simulink model "testmodel"  (R2025b)
settings: Solver=VariableStepAuto  StartTime=0.0  StopTime=2  RelTol=1e-3
values from neighbouring files (symbols this model uses):
  fs = 44100    [model.m]    (also in xgboost.m)
undefined symbols (not defined in the file or in its folder): c
libraries: audiofeatures x6, statsLibrary x3, deeplib x3, audiosources x1
settings Model: Creator=prashanth  LastModifiedBy=prashanth

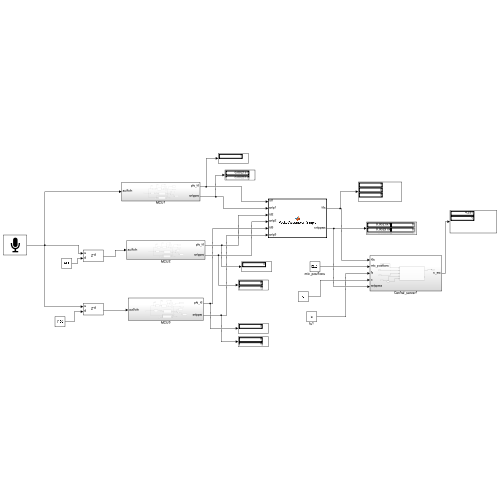
[thumbnail: Simulink's stored preview of the top-level diagram]
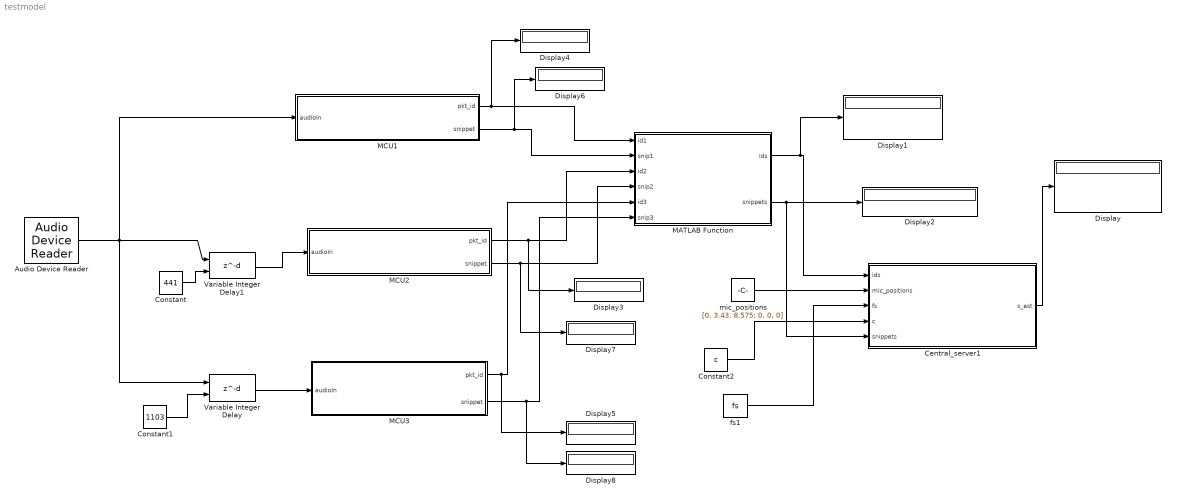
== system testmodel ==
  Audio Device Reader : audiosources/Audio Device Reader  Driver=CoreAudio  Device=Default  SampleRate=44100  NumChannels=1  SamplesPerFrame=44100  BitDepth=16-bit integer  NumBuffers=10  DefaultInputChannelMapping=on  InputChannelMapping=1:2  OutputNumOverrunSamples=off  OutputDataType=double  DriverIdx=5  DeviceWarnFlag=''
  Central_server1 : Subsystem
  Constant : Constant  Value=441
  Constant1 : Constant  Value=1103
  Constant2 : Constant  Value=c
  Display{,1..8} (9 alike) : Display
  MATLAB Function : MATLAB Function  TreatAsAtomicUnit=on
  MCU1 : Subsystem
  MCU2 : Subsystem
  MCU3 : Subsystem
  Variable Integer Delay : Delay  DelayLengthSource=Input port
      settings: InputPortMap=u0,p1
  Variable Integer Delay1 : Delay  DelayLengthSource=Input port
      settings: InputPortMap=u0,p1
  fs1 : Constant  Value=fs
  mic_positions : Constant  Value=[0, 3.43, 8.575; 0, 0, 0]
  wires:
  Audio Device Reader/1 -> MCU1/1(audioIn), Variable Integer Delay1/1, Variable Integer Delay/1
  Variable Integer Delay1/1 -> MCU2/1(audioIn)
  Variable Integer Delay/1 -> MCU3/1(audioIn)
  Constant/1 -> Variable Integer Delay1/2
  Constant1/1 -> Variable Integer Delay/2
  MCU1/1(pkt_id) -> Display4/1, MATLAB Function/1(id1)
  MCU1/2(snippet) -> Display6/1, MATLAB Function/2(snip1)
  MCU3/1(pkt_id) -> Display5/1, MATLAB Function/5(id3)
  MCU3/2(snippet) -> Display8/1, MATLAB Function/6(snip3)
  MATLAB Function/1(ids) -> Display1/1, Central_server1/1(ids)
  fs1/1 -> Central_server1/3(fs)
  mic_positions/1 -> Central_server1/2(mic_positions)
  Constant2/1 -> Central_server1/4(c)
  Central_server1/1(s_est) -> Display/1
  MATLAB Function/2(snippets) -> Central_server1/5(snippets), Display2/1
  MCU2/1(pkt_id) -> Display3/1, MATLAB Function/3(id2)
  MCU2/2(snippet) -> Display7/1, MATLAB Function/4(snip2)

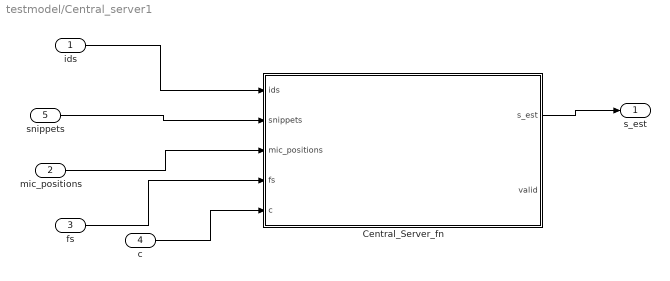
== system testmodel/Central_server1 ==
  ids : Inport
  mic_positions : Inport  Port=2
  fs : Inport  Port=3
  c : Inport  Port=4
  snippets : Inport  Port=5
  Central_Server_fn : MATLAB Function  TreatAsAtomicUnit=on
  s_est : Outport
  wires:
  Central_Server_fn/1(s_est) -> s_est/1
  ids/1 -> Central_Server_fn/1(ids)
  mic_positions/1 -> Central_Server_fn/3(mic_positions)
  fs/1 -> Central_Server_fn/4(fs)
  c/1 -> Central_Server_fn/5(c)
  snippets/1 -> Central_Server_fn/2(snippets)

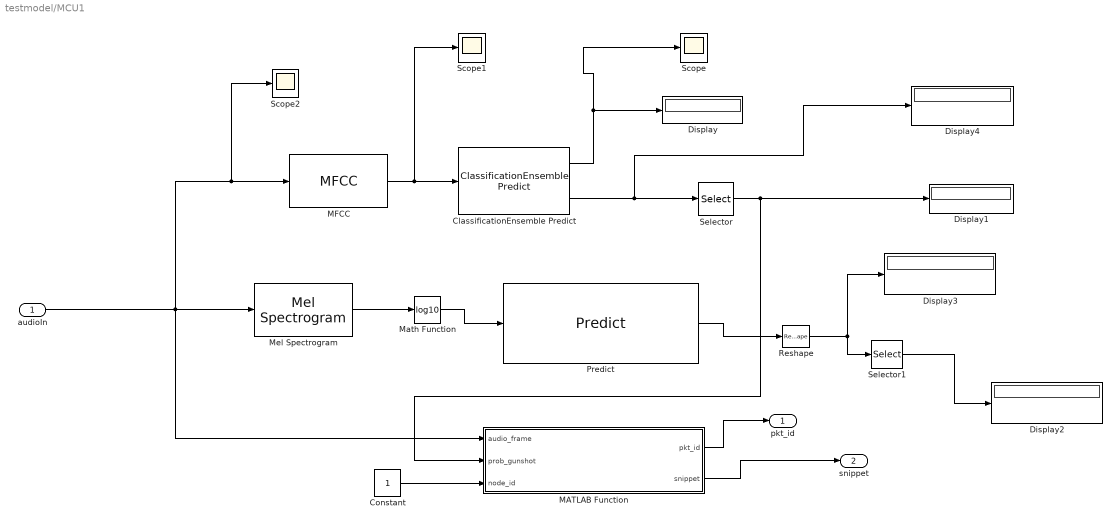
== system testmodel/MCU1 ==
  audioIn : Inport
  ClassificationEnsemble Predict : statsLibrary/Classification/ClassificationEnsemble Predict  TrainedLearner=trainedModel  ShowOutputScore=on  LabelOutMin=[]  LabelOutMax=[]  ScoreOutMin=[]  ScoreOutMax=[]  RawScoreOutMin=[]  RawScoreOutMax=[]  WeakLearnerOutMin=[]  WeakLearnerOutMax=[]  StoredEnumName=trainedModel_enumLabels
  Constant : Constant
  Display{,1..4} (5 alike) : Display
  MATLAB Function : MATLAB Function  TreatAsAtomicUnit=on
  MFCC : audiofeatures/MFCC  WindowParameter=hamming(1024,'periodic')  OverlapLength=512  NumCoeffs=13  Rectification=Logarithm  AppendDelta=on  AppendDeltaDelta=off  DeltaWindowLength=9  NumFeatureVectors=1  NumFeatureVectorOverlap=0  InheritSampleRate=on  SampleRate=44.1e3  NumBands=32  AutoFrequencyRange=on  FrequencyRange=[0, 22050]  FilterBankDesignDomain=linear  FilterBankNormalization=bandwidth  MelStyle=oshaughnessy  WindowNormalization=on  SpectrumType=power  AutoFFTLength=on  FFTLength=1024
  Math Function : Math  Operator=log10
  Mel Spectrogram : audiofeatures/Mel Spectrogram  FrequencyScale=mel  AutoNumBands=off  NumBands=32  AutoFrequencyRange=on  FrequencyRange=[0, 22050]  FilterBankDesignDomain=linear  FilterBankNormalization=bandwidth  MelStyle=oshaughnessy  OutputFrequencyVector=off  WindowParameter=hamming(1024,'periodic')  WindowNormalization=on  OverlapLength=512  AutoFFTLength=on  FFTLength=1024  SpectrumType=magnitude  ApplyLog=off  NumHops=85  NumHopsOverlap=0  InheritSampleRate=on  SampleRate=44.1e3
  Predict : deeplib/Predict  Network=Network from MAT-file  NetworkFunction=squeezenet  NetworkFilePath=/Users/prashanth/Desktop/karthik/gunshotCNN.mat  MiniBatchSize=128  InputDataFormats={'',''}  Predictions=off  Activations={'softmax'}  ForceInterpretedSim=off  EnableDLNetwork=on  LastKnownNetworkFilePath=''  LastKnownNetworkTimeStamp=''
  Reshape : Reshape
  Scope : Scope
      settings: ActiveDisplayYMinimum=-1  ActiveDisplayYMaximum=1
  Scope1 : Scope
      settings: ActiveDisplayYMinimum=-2027.6320329799446  ActiveDisplayYMaximum=845.22597661163
  Scope2 : Scope
      settings: ActiveDisplayYMinimum=-0.30791958580274859  ActiveDisplayYMaximum=0.10660759871682185  DataLoggingVariableName=ScopeData2
  Selector : Selector  InputPortWidth=2  IndexOptions=Index vector (dialog)  Indices=1  OutputSizes=1
  Selector1 : Selector  InputPortWidth=2  IndexOptions=Index vector (dialog)  Indices=1  OutputSizes=1
  pkt_id : Outport
  snippet : Outport  Port=2
  wires:
  Selector/1 -> MATLAB Function/2(prob_gunshot), Display1/1
  Reshape/1 -> Selector1/1, Display3/1
  MFCC/1 -> Scope1/1, ClassificationEnsemble Predict/1
  Predict/1 -> Reshape/1
  Mel Spectrogram/1 -> Math Function/1
  Selector1/1 -> Display2/1
  Math Function/1 -> Predict/1
  audioIn/1 -> MATLAB Function/1(audio_frame), Mel Spectrogram/1, MFCC/1, Scope2/1
  ClassificationEnsemble Predict/2 -> Display4/1, Selector/1
  ClassificationEnsemble Predict/1 -> Scope/1, Display/1
  Constant/1 -> MATLAB Function/3(node_id)
  MATLAB Function/1(pkt_id) -> pkt_id/1
  MATLAB Function/2(snippet) -> snippet/1

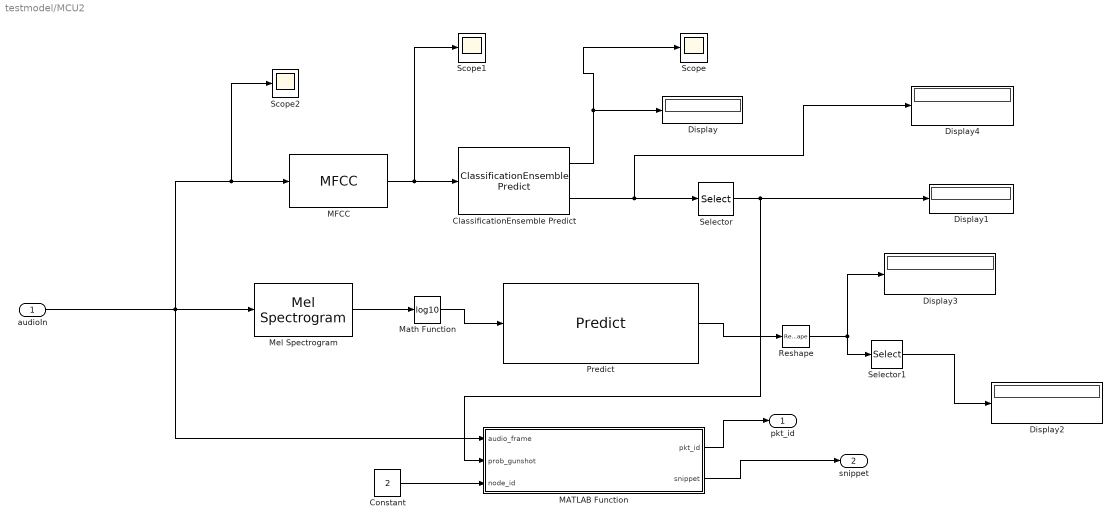
== system testmodel/MCU2 ==
  audioIn : Inport
  ClassificationEnsemble Predict : statsLibrary/Classification/ClassificationEnsemble Predict  TrainedLearner=trainedModel  ShowOutputScore=on  LabelOutMin=[]  LabelOutMax=[]  ScoreOutMin=[]  ScoreOutMax=[]  RawScoreOutMin=[]  RawScoreOutMax=[]  WeakLearnerOutMin=[]  WeakLearnerOutMax=[]  StoredEnumName=trainedModel_enumLabels
  Constant : Constant  Value=2
  Display{,1..4} (5 alike) : Display
  MATLAB Function : MATLAB Function  TreatAsAtomicUnit=on
  MFCC : audiofeatures/MFCC  WindowParameter=hamming(1024,'periodic')  OverlapLength=512  NumCoeffs=13  Rectification=Logarithm  AppendDelta=on  AppendDeltaDelta=off  DeltaWindowLength=9  NumFeatureVectors=1  NumFeatureVectorOverlap=0  InheritSampleRate=on  SampleRate=44.1e3  NumBands=32  AutoFrequencyRange=on  FrequencyRange=[0, 22050]  FilterBankDesignDomain=linear  FilterBankNormalization=bandwidth  MelStyle=oshaughnessy  WindowNormalization=on  SpectrumType=power  AutoFFTLength=on  FFTLength=1024
  Math Function : Math  Operator=log10
  Mel Spectrogram : audiofeatures/Mel Spectrogram  FrequencyScale=mel  AutoNumBands=off  NumBands=32  AutoFrequencyRange=on  FrequencyRange=[0, 22050]  FilterBankDesignDomain=linear  FilterBankNormalization=bandwidth  MelStyle=oshaughnessy  OutputFrequencyVector=off  WindowParameter=hamming(1024,'periodic')  WindowNormalization=on  OverlapLength=512  AutoFFTLength=on  FFTLength=1024  SpectrumType=magnitude  ApplyLog=off  NumHops=85  NumHopsOverlap=0  InheritSampleRate=on  SampleRate=44.1e3
  Predict : deeplib/Predict  Network=Network from MAT-file  NetworkFunction=squeezenet  NetworkFilePath=/Users/prashanth/Desktop/karthik/gunshotCNN.mat  MiniBatchSize=128  InputDataFormats={'',''}  Predictions=off  Activations={'softmax'}  ForceInterpretedSim=off  EnableDLNetwork=on  LastKnownNetworkFilePath=''  LastKnownNetworkTimeStamp=''
  Reshape : Reshape
  Scope : Scope
      settings: ActiveDisplayYMinimum=0.875  ActiveDisplayYMaximum=2.125  DataLoggingVariableName=ScopeData3
  Scope1 : Scope
      settings: ActiveDisplayYMinimum=-2027.6320329799446  ActiveDisplayYMaximum=845.22597661163  DataLoggingVariableName=ScopeData4
  Scope2 : Scope
      settings: ActiveDisplayYMinimum=-0.30791958580274859  ActiveDisplayYMaximum=0.10660759871682185  DataLoggingVariableName=ScopeData5
  Selector : Selector  InputPortWidth=2  IndexOptions=Index vector (dialog)  Indices=1  OutputSizes=1
  Selector1 : Selector  InputPortWidth=2  IndexOptions=Index vector (dialog)  Indices=1  OutputSizes=1
  pkt_id : Outport
  snippet : Outport  Port=2
  wires:
  Mel Spectrogram/1 -> Math Function/1
  Math Function/1 -> Predict/1
  ClassificationEnsemble Predict/2 -> Display4/1, Selector/1
  Constant/1 -> MATLAB Function/3(node_id)
  ClassificationEnsemble Predict/1 -> Scope/1, Display/1
  MATLAB Function/1(pkt_id) -> pkt_id/1
  Predict/1 -> Reshape/1
  Selector1/1 -> Display2/1
  Reshape/1 -> Selector1/1, Display3/1
  MFCC/1 -> Scope1/1, ClassificationEnsemble Predict/1
  MATLAB Function/2(snippet) -> snippet/1
  Selector/1 -> MATLAB Function/2(prob_gunshot), Display1/1
  audioIn/1 -> MATLAB Function/1(audio_frame), Mel Spectrogram/1, MFCC/1, Scope2/1

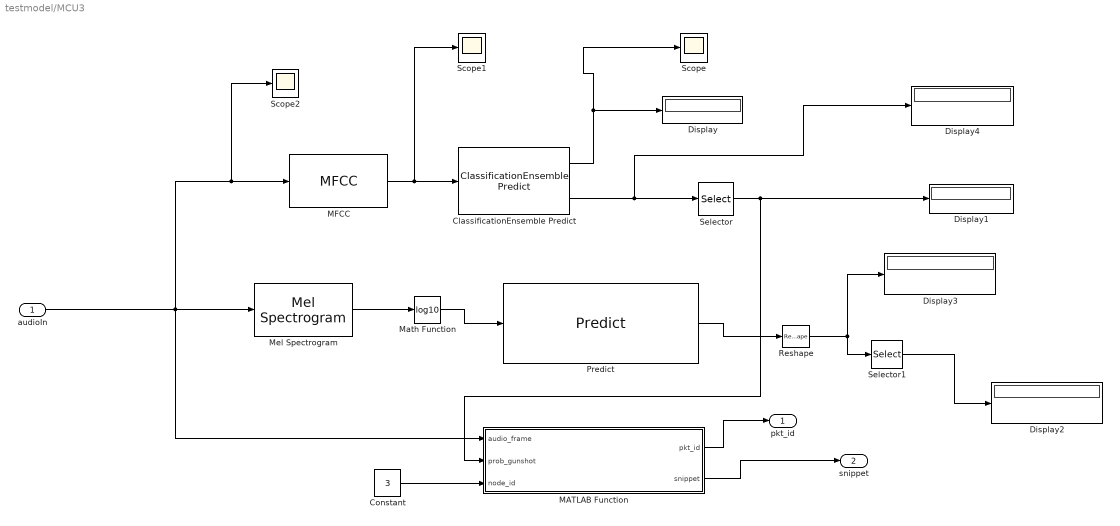
== system testmodel/MCU3 ==
  audioIn : Inport
  ClassificationEnsemble Predict : statsLibrary/Classification/ClassificationEnsemble Predict  TrainedLearner=trainedModel  ShowOutputScore=on  LabelOutMin=[]  LabelOutMax=[]  ScoreOutMin=[]  ScoreOutMax=[]  RawScoreOutMin=[]  RawScoreOutMax=[]  WeakLearnerOutMin=[]  WeakLearnerOutMax=[]  StoredEnumName=trainedModel_enumLabels
  Constant : Constant  Value=3
  Display{,1..4} (5 alike) : Display
  MATLAB Function : MATLAB Function  TreatAsAtomicUnit=on
  MFCC : audiofeatures/MFCC  WindowParameter=hamming(1024,'periodic')  OverlapLength=512  NumCoeffs=13  Rectification=Logarithm  AppendDelta=on  AppendDeltaDelta=off  DeltaWindowLength=9  NumFeatureVectors=1  NumFeatureVectorOverlap=0  InheritSampleRate=on  SampleRate=44.1e3  NumBands=32  AutoFrequencyRange=on  FrequencyRange=[0, 22050]  FilterBankDesignDomain=linear  FilterBankNormalization=bandwidth  MelStyle=oshaughnessy  WindowNormalization=on  SpectrumType=power  AutoFFTLength=on  FFTLength=1024
  Math Function : Math  Operator=log10
  Mel Spectrogram : audiofeatures/Mel Spectrogram  FrequencyScale=mel  AutoNumBands=off  NumBands=32  AutoFrequencyRange=on  FrequencyRange=[0, 22050]  FilterBankDesignDomain=linear  FilterBankNormalization=bandwidth  MelStyle=oshaughnessy  OutputFrequencyVector=off  WindowParameter=hamming(1024,'periodic')  WindowNormalization=on  OverlapLength=512  AutoFFTLength=on  FFTLength=1024  SpectrumType=magnitude  ApplyLog=off  NumHops=85  NumHopsOverlap=0  InheritSampleRate=on  SampleRate=44.1e3
  Predict : deeplib/Predict  Network=Network from MAT-file  NetworkFunction=squeezenet  NetworkFilePath=/Users/prashanth/Desktop/karthik/gunshotCNN.mat  MiniBatchSize=128  InputDataFormats={'',''}  Predictions=off  Activations={'softmax'}  ForceInterpretedSim=off  EnableDLNetwork=on  LastKnownNetworkFilePath=''  LastKnownNetworkTimeStamp=''
  Reshape : Reshape
  Scope : Scope
      settings: ActiveDisplayYMinimum=0.875  ActiveDisplayYMaximum=2.125  DataLoggingVariableName=ScopeData6
  Scope1 : Scope
      settings: ActiveDisplayYMinimum=-2027.6320329799446  ActiveDisplayYMaximum=845.22597661163  DataLoggingVariableName=ScopeData7
  Scope2 : Scope
      settings: ActiveDisplayYMinimum=-0.30791958580274859  ActiveDisplayYMaximum=0.10660759871682185  DataLoggingVariableName=ScopeData8
  Selector : Selector  InputPortWidth=2  IndexOptions=Index vector (dialog)  Indices=1  OutputSizes=1
  Selector1 : Selector  InputPortWidth=2  IndexOptions=Index vector (dialog)  Indices=1  OutputSizes=1
  pkt_id : Outport
  snippet : Outport  Port=2
  wires:
  Mel Spectrogram/1 -> Math Function/1
  Math Function/1 -> Predict/1
  ClassificationEnsemble Predict/2 -> Display4/1, Selector/1
  Constant/1 -> MATLAB Function/3(node_id)
  ClassificationEnsemble Predict/1 -> Scope/1, Display/1
  MATLAB Function/1(pkt_id) -> pkt_id/1
  Predict/1 -> Reshape/1
  Selector1/1 -> Display2/1
  Reshape/1 -> Selector1/1, Display3/1
  MFCC/1 -> Scope1/1, ClassificationEnsemble Predict/1
  MATLAB Function/2(snippet) -> snippet/1
  Selector/1 -> MATLAB Function/2(prob_gunshot), Display1/1
  audioIn/1 -> MATLAB Function/1(audio_frame), Mel Spectrogram/1, MFCC/1, Scope2/1

== matlab function testmodel/MCU1/MATLAB Function ==
  data: audio_frame input; pkt_id output; prob_gunshot input; node_id input; snippet output
function [pkt_id, snippet] = Gatekeeper(audio_frame, prob_gunshot, node_id)
    %#codegen
    % 1. Setup Fixed Output
    L = 512; 
    snippet = zeros(L, 1); % Defines snippet as FIXED [512 x 1]
    pkt_id = -1;
    
    % 2. Threshold Check
    if prob_gunshot > 0.2
        
        % 3. Find the Peak
        [~, peak_idx] = max(abs(audio_frame));
        
        % 4. Calculate Indices
        start_idx = peak_idx - floor(L/2);
        end_idx   = start_idx + L - 1;
        
        % 5. Handle Edge Cases (Clamp to frame boundaries)
        frame_len = length(audio_frame);
        
        % If peak is too close to the start
        if start_idx < 1
            start_idx = 1;
            end_idx = min(L, frame_len);
        end
        
        % If peak is too close to the end
        if end_idx > frame_len
            end_idx = frame_len;
            start_idx = max(1, frame_len - L + 1);
        end
        
        % 6. SAFE ASSIGNMENT (The Fix)
        % We calculate the exact length of data we are about to copy
        data_len = end_idx - start_idx + 1;
        
        % We manually copy the data into the first 'data_len' slots of snippet.
        % This PRESERVES the fixed size of the 'snippet' variable.
        if data_len > 0
            snippet(1:data_len) = audio_frame(start_idx:end_idx);
        end
        
        pkt_id = node_id;
    end
end

== matlab function testmodel/MCU2/MATLAB Function ==
  data: audio_frame input; pkt_id output; prob_gunshot input; node_id input; snippet output
function [pkt_id, snippet] = Gatekeeper(audio_frame, prob_gunshot, node_id)
    %#codegen
    % 1. Setup Fixed Output
    L = 512; 
    snippet = zeros(L, 1); % Defines snippet as FIXED [512 x 1]
    pkt_id = -1;
    
    % 2. Threshold Check
    if prob_gunshot > 0.2
        
        % 3. Find the Peak
        [~, peak_idx] = max(abs(audio_frame));
        
        % 4. Calculate Indices
        start_idx = peak_idx - floor(L/2);
        end_idx   = start_idx + L - 1;
        
        % 5. Handle Edge Cases (Clamp to frame boundaries)
        frame_len = length(audio_frame);
        
        % If peak is too close to the start
        if start_idx < 1
            start_idx = 1;
            end_idx = min(L, frame_len);
        end
        
        % If peak is too close to the end
        if end_idx > frame_len
            end_idx = frame_len;
            start_idx = max(1, frame_len - L + 1);
        end
        
        % 6. SAFE ASSIGNMENT (The Fix)
        % We calculate the exact length of data we are about to copy
        data_len = end_idx - start_idx + 1;
        
        % We manually copy the data into the first 'data_len' slots of snippet.
        % This PRESERVES the fixed size of the 'snippet' variable.
        if data_len > 0
            snippet(1:data_len) = audio_frame(start_idx:end_idx);
        end
        
        pkt_id = node_id;
    end
end

== matlab function testmodel/MCU3/MATLAB Function ==
  data: audio_frame input; pkt_id output; prob_gunshot input; node_id input; snippet output
function [pkt_id, snippet] = Gatekeeper(audio_frame, prob_gunshot, node_id)
    %#codegen
    % 1. Setup Fixed Output
    L = 512; 
    snippet = zeros(L, 1); % Defines snippet as FIXED [512 x 1]
    pkt_id = -1;
    
    % 2. Threshold Check
    if prob_gunshot > 0.2
        
        % 3. Find the Peak
        [~, peak_idx] = max(abs(audio_frame));
        
        % 4. Calculate Indices
        start_idx = peak_idx - floor(L/2);
        end_idx   = start_idx + L - 1;
        
        % 5. Handle Edge Cases (Clamp to frame boundaries)
        frame_len = length(audio_frame);
        
        % If peak is too close to the start
        if start_idx < 1
            start_idx = 1;
            end_idx = min(L, frame_len);
        end
        
        % If peak is too close to the end
        if end_idx > frame_len
            end_idx = frame_len;
            start_idx = max(1, frame_len - L + 1);
        end
        
        % 6. SAFE ASSIGNMENT (The Fix)
        % We calculate the exact length of data we are about to copy
        data_len = end_idx - start_idx + 1;
        
        % We manually copy the data into the first 'data_len' slots of snippet.
        % This PRESERVES the fixed size of the 'snippet' variable.
        if data_len > 0
            snippet(1:data_len) = audio_frame(start_idx:end_idx);
        end
        
        pkt_id = node_id;
    end
end

== matlab function testmodel/MATLAB Function ==
  data: id1 input; ids output; snip1 input; id2 input; snip2 input; id3 input; snip3 input; snippets output
function [ids, snippets] = PacketAssembler_Simple(id1, snip1, id2, snip2, id3, snip3)
    %#codegen
    % Simplified Assembler: Takes data from 3 Smart MCUs and bundles it
    % for the Central Server.
    
    % 1. Bundle IDs into a [3x1] vector
    ids = [id1; id2; id3];
    
    % 2. Bundle Snippets into a [L x 3] matrix
    % Columns = Mic 1, Mic 2, Mic 3
    L = 512; % Must match your MCU snippet size
    snippets = zeros(L, 3);
    
    snippets(:, 1) = snip1;
    snippets(:, 2) = snip2;
    snippets(:, 3) = snip3;
end

== matlab function testmodel/Central_server1/Central_Server_fn ==
  data: ids input; s_est output; snippets input; mic_positions input; fs input; c input; valid output
function [s_est, valid] = Central_Server_fn(ids, snippets, mic_positions, fs, c)
% Central_Server_fn - GCC-PHAT based TDOA localization
% Inputs:
%   ids          : [N x 1] node ids (double)
%   snippets     : [L x N] snippet columns, each column is snippet from mic j
%   mic_positions: [2 x N] mic coordinates (meters)
%   fs           : sampling rate (Hz)
%   c            : speed of sound (m/s)
% Outputs:
%   s_est        : [2 x 1] estimated source location (m)
%   valid        : logical/double true if estimate computed

%#codegen
valid = false;
s_est = zeros(2,1);

% basic checks
% 1. Check for empty or wrong size
if isempty(ids) || isempty(snippets) || size(snippets,2) < 3
    valid = false;
    return;
end

% 2. CRITICAL FIX: Check if IDs are valid (-1 means no detection)
if any(ids < 0)
    % If ANY node reports "No Gunshot", we cannot triangulate.
    s_est = [0; 0]; 
    valid = false;
    return;
end

% 3. Check for silence (all zeros)
if sum(abs(snippets(:))) == 0
    s_est = [0; 0];
    valid = false;
    return;
end
N = size(snippets,2);
L = size(snippets,1);

% choose reference mic as column 1
ref = 1;

% Pre-allocate tdoa (seconds) vector for pairs ref->j
tdoa_meas = zeros(N-1,1);
pair_idx = 0;

% FFT length for cross-correlation (next pow of 2 >= 2*L)
nfft = 2^nextpow2(2*L);

% compute GCC-PHAT between ref and each other mic
Xref = fft(snippets(:,ref), nfft);
for j = 1:N
    if j == ref, continue; end
    pair_idx = pair_idx + 1;
    Xj = fft(snippets(:,j), nfft);
    R = Xref .* conj(Xj);
    % PHAT weight
    R = R ./ (abs(R) + eps);
    cc = ifft(R);
    % cc is length nfft, find peak and refine by parabolic interpolation
    % shift cross-corr so lags: -nfft/2..nfft/2-1
    ccmag = abs(cc);
    [~, Imax] = max(ccmag);
    % convert to zero-based index
    k = Imax - 1;
    % handle wrapping: convert index to signed lag in samples
    if k <= nfft/2 - 1
        lag = k;
    else
        lag = k - nfft;
    end
    % parabolic interpolation around Imax (use modular indexing)
    left = mod(Imax-2, nfft) + 1;
    right = mod(Imax, nfft) + 1;
    y1 = ccmag(left); y2 = ccmag(Imax); y3 = ccmag(right);
    denom = (y1 - 2*y2 + y3);
    if abs(denom) < eps
        delta = 0.0;
    else
        delta = 0.5 * (y1 - y3) / denom;   % fractional offset (samples)
    end
    lag_corrected = double(lag) + double(delta);
    % convert lag (samples) to time (seconds) t_ref - t_j
    tdoa_meas(pair_idx) = -lag_corrected / double(fs); 
    % NOTE: we used lag as index of cc = correlation ref vs j, and defined tdoa as (t_j - t_ref).
    % sign convention chosen so (di - dj)/c = tdoa_ref_j, solver below expects (di-dj)/c = tvec(i)-tvec(j)
end

% Build pairs array for solver: we will create pairs between mics [1..N] using ref as anchor
% Convert tdoa_meas to pairwise format consistent with solver: for i=ref and j others:
pairs = zeros(N-1,2);
for k = 1:(N-1)
    pairs(k,1) = ref;
    pairs(k,2) = k+1;
end

% initial guess: centroid of microphone positions
s = mean(mic_positions,2);

% Gauss-Newton solve (use same residual model as earlier)
for iter = 1:10
    m = size(pairs,1);
    r = zeros(m,1); J = zeros(m,2);
    for k = 1:m
        i = pairs(k,1);
        j = pairs(k,2);
        pi = mic_positions(:,i);
        pj = mic_positions(:,j);
        di = norm(s - pi); dj = norm(s - pj);
        if di == 0, di = 1e-6; end
        if dj == 0, dj = 1e-6; end
        % predicted TDOA (seconds) = (di - dj) / c
        pred = (di - dj) / c;
        r(k) = pred - tdoa_meas(k);
        J(k,1) = ((s(1)-pi(1))/di - (s(1)-pj(1))/dj) / c;
        J(k,2) = ((s(2)-pi(2))/di - (s(2)-pj(2))/dj) / c;
    end
    H = J' * J + 1e-6 * eye(2);
    delta = H \ (J' * r);
    s = s - delta;
    if norm(delta) < 1e-6
        break;
    end
end

s_est = s;
valid = true;
end
